simulink subsystem "GantryRobotSubsystem"  (R2024a)
settings: Solver=VariableStepAuto  StartTime=0.0  StopTime=10.0  RelTol=1e-3
model mask{DOF=3DOF, configAxis=XYZ, heightColumn=0.4, widthColumn=0.05, positionColumn1=[-0.5,-0.5,0], positionColumn2=[0.5,-0.5,0], positionColumn3=[-0.5,0.5,0], positionColumn4=[0.5,0.5,0], systemGuideX=Rail-block, strokeXMax=1, widthGuideX=0.05, diaScrewX=0.05, widthXMount=0.1, typeInertiaGuideX=Calculate from Geometry, densityGuideX=2700, massGuideX=0.1, COMGuideX=[0 0 0], MOIGuideX=[0.01 0.01 0.01], POIGuideX=[0 0 0], typeInertiaCarriageX=Calculate from Geometry, densityCarriageX=2700, massCarriageX=0.1, COMCarriageX=[0 0 0], MOICarriageX=[0.01 0.01 0.01], POICarriageX=[0 0 0], colorGuideX=[0.7 0.6 0.4], colorCarriageX=[0.5 0.5 0.9], systemGuideY=Rail-block, strokeYMax=1, widthGuideY=0.05, diaScrewY=0.05, widthYMount=0.05, typeInertiaGuideY=Calculate from Geometry, densityGuideY=2700, massGuideY=0.1, COMGuideY=[0 0 0], MOIGuideY=[0.01 0.01 0.01], POIGuideY=[0 0 0], typeInertiaCarriageY=Calculate from Geometry, densityCarriageY=2700, massCarriageY=0.1, COMCarriageY=[0 0 0], MOICarriageY=[0.01 0.01 0.01], POICarriageY=[0 0 0], colorGuideY=[0.7 0.6 0.4], colorCarriageY=[0.5 0.5 0.9], systemGuideZ=Rail-block, strokeZMax=1, widthGuideZ=0.05, diaScrewZ=0.05, shiftZAxisDown=0.02, widthZMount=0.05, typeInertiaGuideZ=Calculate from Geometry, densityGuideZ=2700, massGuideZ=0.1, COMGuideZ=[0 0 0], MOIGuideZ=[0.01 0.01 0.01], POIGuideZ=[0 0 0], typeInertiaCarriageZ=Calculate from Geometry, densityCarriageZ=2700, massCarriageZ=0.1, COMCarriageZ=[0 0 0], MOICarriageZ=[0.01 0.01 0.01], POICarriageZ=[0 0 0], colorGuideZ=[0.7 0.6 0.4], colorCarriageZ=[0.5 0.5 0.9]}
  mask prompts: DOF "Degrees of freedom"; configAxis "Axis configurations"; heightColumn "Column height (m)"; widthColumn "Column width (m)"; positionColumn1 "Column 1 position (m)"; positionColumn2 "Column 2 position (m)"; positionColumn3 "Column 3 position (m)"; positionColumn4 "Column 4 position (m)"; systemGuideX "Guide system"; strokeXMax "Maximum stroke (m)"; widthGuideX "Guide width (m)"; diaScrewX "Screw diameter (m)"; widthXMount "Mount width (m)"; typeInertiaGuideX "Inertia type"; densityGuideX "Density (kg/m^3)"; massGuideX "Mass (kg)"; COMGuideX "Center of mass (m)"; MOIGuideX "Moments of inertia (kg*m^2)"; POIGuideX "Products of inertia (kg*m^2)"; typeInertiaCarriageX "Inertia type"; densityCarriageX "Density (kg/m^3)"; massCarriageX "Mass (kg)"; COMCarriageX "Center of mass (m)"; MOICarriageX "Moments of inertia (kg*m^2)"; POICarriageX "Products of inertia (kg*m^2)"; colorGuideX "Linear guide color"; colorCarriageX "Carriage color"; systemGuideY "Guide system"; strokeYMax "Maximum stroke (m)"; widthGuideY "Guide width (m)"; diaScrewY "Screw diameter (m)"; widthYMount "Mount width (m)"; typeInertiaGuideY "Inertia type"; densityGuideY "Density (kg/m^3)"; massGuideY "Mass (kg)"; COMGuideY "Center of mass (m)"; MOIGuideY "Moments of inertia (kg*m^2)"; POIGuideY "Products of inertia (kg*m^2)"; typeInertiaCarriageY "Inertia type"; densityCarriageY "Density (kg/m^3)"; massCarriageY "Mass (kg)"; COMCarriageY "Center of mass (m)"; MOICarriageY "Moments of inertia (kg*m^2)"; POICarriageY "Products of inertia (kg*m^2)"; colorGuideY "Linear guide color"; colorCarriageY "Carriage color"; systemGuideZ "Guide system"; strokeZMax "Maximum stroke (m)"; widthGuideZ "Guide width (m)"; diaScrewZ "Screw diameter (m)"; shiftZAxisDown "Downward shift of Z-axis (m)"; widthZMount "Mount width (m)"; typeInertiaGuideZ "Inertia type"; densityGuideZ "Density (kg/m^3)"; massGuideZ "Mass (kg)"; COMGuideZ "Center of mass (m)"; MOIGuideZ "Moments of inertia (kg*m^2)"; POIGuideZ "Products of inertia (kg*m^2)"; typeInertiaCarriageZ "Inertia type"; densityCarriageZ "Density (kg/m^3)"; massCarriageZ "Mass (kg)"; COMCarriageZ "Center of mass (m)"; MOICarriageZ "Moments of inertia (kg*m^2)"; POICarriageZ "Products of inertia (kg*m^2)"; colorGuideZ "Linear guide color"; colorCarriageZ "Carriage color"
undefined symbols (not defined in the file): X, Y, Z
libraries: sm_lib x92, CartesianLib x46, nesl_utility x38
(part 4 of 4)

== system GantryRobotSubsystem/GantryRobotVariant/XYZR Gantry/Y-Axis Unit ==
  PS-Simulink Converter : nesl_utility/PS-Simulink Converter  PhysicalDomain=network_engine_domain  SubClassName=ps_output  LeftPortType=input  RightPortType=output  PseudoPeriodic=off  Frequencies=[]  VectorFormat=inherit  Unit=inherit  AffineConversion=off
  PS-Simulink Converter1 : nesl_utility/PS-Simulink Converter  PhysicalDomain=network_engine_domain  SubClassName=ps_output  LeftPortType=input  RightPortType=output  PseudoPeriodic=off  Frequencies=[]  VectorFormat=inherit  Unit=inherit  AffineConversion=off
  PS-Simulink Converter2 : nesl_utility/PS-Simulink Converter  PhysicalDomain=network_engine_domain  SubClassName=ps_output  LeftPortType=input  RightPortType=output  PseudoPeriodic=off  Frequencies=[]  VectorFormat=inherit  Unit=inherit  AffineConversion=off
  Prismatic Joint2 : sm_lib/Joints/Prismatic Joint  JointMode=Normal  CompositeWrenchDir=FollowerOnBase  CompositeWrenchFrame=BaseFrame  SenseConstraintForce=off  SenseConstraintTorque=off  SenseTotalForce=off  SenseTotalTorque=off  PositionTargetSpecify=off  PositionTargetPriority=High  PositionTargetValue=0  PositionTargetValueUnits=m  VelocityTargetSpecify=off  VelocityTargetPriority=High  VelocityTargetValue=0  VelocityTargetValueUnits=m/s  EquilibriumPosition=0  EquilibriumPositionUnits=m  SpringStiffness=0  SpringStiffnessUnits=N/m  DampingCoefficient=0  DampingCoefficientUnits=N/(m/s)  LowerLimitSpecify=on  LowerLimitBound=-0.5*strokeYMax  LowerLimitBoundUnits=m  LowerLimitStiffness=1e6  LowerLimitStiffnessUnits=N/m  LowerLimitDamping=1e3  LowerLimitDampingUnits=N/(m/s)  LowerLimitTransitionRegionWidth=1e-4  LowerLimitTransitionRegionWidthUnits=m  UpperLimitSpecify=on  UpperLimitBound=0.5*strokeYMax  UpperLimitBoundUnits=m  UpperLimitStiffness=1e6  UpperLimitStiffnessUnits=N/m  UpperLimitDamping=1e3  UpperLimitDampingUnits=N/(m/s)  UpperLimitTransitionRegionWidth=1e-4  UpperLimitTransitionRegionWidthUnits=m  TorqueActuationMode=InputTorque  MotionActuationMode=ComputedMotion  SensePosition=on  SenseVelocity=on  SenseAcceleration=on  SenseTorqueForce=off  SenseLowerLimitTorqueForce=off  SenseUpperLimitTorqueForce=off
  Rigid Transform1 : sm_lib/Frames and Transforms/Rigid Transform  RotationMethod=None  FollAlignAxisA=+X  BaseAlignAxisA=+Y  FollAlignAxisB=+Y  BaseAlignAxisB=+Z  RotationStandardAxis=+Z  RotationAngle=0  RotationAngleUnits=deg  RotationArbitraryAxis=[0 0 1]  RotationSequenceAxes=BaseAxes  RotationSequence=XYZ  RotationSequenceAngles=[0 0 0]  RotationSequenceAnglesUnits=deg  RotationMatrix=[1 0 0;0 1 0;0 0 1]  Quaternion=[1 0 0 0]  TranslationMethod=StandardAxis  TranslationCartesianOffset=[0 0 0]  TranslationCartesianOffsetUnits=m  TranslationStandardAxis=+Y  TranslationStandardOffset=-positionColumn1(2)  TranslationStandardOffsetUnits=m  TranslationROffset=0  TranslationROffsetUnits=m  TranslationThetaOffset=0  TranslationThetaOffsetUnits=deg  TranslationZOffset=0  TranslationZOffsetUnits=m
  Rigid Transform2 : sm_lib/Frames and Transforms/Rigid Transform  RotationMethod=None  FollAlignAxisA=+X  BaseAlignAxisA=+Y  FollAlignAxisB=+Y  BaseAlignAxisB=+Z  RotationStandardAxis=+Z  RotationAngle=0  RotationAngleUnits=deg  RotationArbitraryAxis=[0 0 1]  RotationSequenceAxes=BaseAxes  RotationSequence=XYZ  RotationSequenceAngles=[0 0 0]  RotationSequenceAnglesUnits=deg  RotationMatrix=[1 0 0;0 1 0;0 0 1]  Quaternion=[1 0 0 0]  TranslationMethod=StandardAxis  TranslationCartesianOffset=[0 0 0]  TranslationCartesianOffsetUnits=m  TranslationStandardAxis=+Y  TranslationStandardOffset=positionColumn2(2)  TranslationStandardOffsetUnits=m  TranslationROffset=0  TranslationROffsetUnits=m  TranslationThetaOffset=0  TranslationThetaOffsetUnits=deg  TranslationZOffset=0  TranslationZOffsetUnits=m
  Rigid Transform3 : sm_lib/Frames and Transforms/Rigid Transform  RotationMethod=StandardAxis  FollAlignAxisA=+X  BaseAlignAxisA=+Y  FollAlignAxisB=+Y  BaseAlignAxisB=+Z  RotationStandardAxis=+X  RotationAngle=-90  RotationAngleUnits=deg  RotationArbitraryAxis=[0 0 1]  RotationSequenceAxes=FollowerAxes  RotationSequence=XYX  RotationSequenceAngles=[0 0 0]  RotationSequenceAnglesUnits=deg  RotationMatrix=[1 0 0;0 1 0;0 0 1]  Quaternion=[1 0 0 0]  TranslationMethod=None  TranslationCartesianOffset=[0 0 0]  TranslationCartesianOffsetUnits=m  TranslationStandardAxis=+Z  TranslationStandardOffset=0  TranslationStandardOffsetUnits=m  TranslationROffset=0  TranslationROffsetUnits=m  TranslationThetaOffset=0  TranslationThetaOffsetUnits=deg  TranslationZOffset=0  TranslationZOffsetUnits=m
  Rigid Transform4 : sm_lib/Frames and Transforms/Rigid Transform  RotationMethod=StandardAxis  FollAlignAxisA=+X  BaseAlignAxisA=+Y  FollAlignAxisB=+Y  BaseAlignAxisB=+Z  RotationStandardAxis=+X  RotationAngle=90  RotationAngleUnits=deg  RotationArbitraryAxis=[0 0 1]  RotationSequenceAxes=FollowerAxes  RotationSequence=XYX  RotationSequenceAngles=[0 0 0]  RotationSequenceAnglesUnits=deg  RotationMatrix=[1 0 0;0 1 0;0 0 1]  Quaternion=[1 0 0 0]  TranslationMethod=None  TranslationCartesianOffset=[0 0 0]  TranslationCartesianOffsetUnits=m  TranslationStandardAxis=+Z  TranslationStandardOffset=0  TranslationStandardOffsetUnits=m  TranslationROffset=0  TranslationROffsetUnits=m  TranslationThetaOffset=0  TranslationThetaOffsetUnits=deg  TranslationZOffset=0  TranslationZOffsetUnits=m
  Y-Axis Linear Stage : CartesianLib/Linear Stage  systemGuide=Rail-block  axisGuide=Y-axis  stroke=1  widthRail=0.05  diaScrew=0.05  typeInertiaGuide=Calculate from Geometry  densityGuide=2700  massGuide=0.1  CMGuide=[0 0 0]  MOIGuide=[0.01 0.01 0.01]  POIGuide=[0 0 0]  typeInertiaCarriage=Calculate from Geometry  densityCarriage=2700  massCarriage=0.1  CMCarriage=[0 0 0]  MOICarriage=[0.01 0.01 0.01]  POICarriage=[0 0 0]  colorGuide=colorGuideY  colorCarriage=colorCarriageY
  YA : PMIOPort  Side=Left
  F : PMIOPort  Port=2  Side=Left
  B1 : PMIOPort  Port=3  Side=Right
  B2 : PMIOPort  Port=4  Side=Right
  Out Bus Element : Outport  PortName=YS  Element=Yp (m)
  BusElementOut : Outport  PortName=YS  Element=Yv (m/s)
  BusElementOut1 : Outport  PortName=YS  Element=Ya (m^2/s)
  wires:
  PS-Simulink Converter/1 -> Out Bus Element/1
  PS-Simulink Converter2/1 -> BusElementOut1/1
  PS-Simulink Converter1/1 -> BusElementOut/1
  connections:
  Prismatic Joint2/RConn4 -- PS-Simulink Converter2/LConn1
  Prismatic Joint2/RConn2 -- PS-Simulink Converter/LConn1
  Prismatic Joint2/RConn3 -- PS-Simulink Converter1/LConn1
  Rigid Transform2/LConn1 -- B2/RConn1
  F/RConn1 -- Y-Axis Linear Stage/LConn1
  Rigid Transform1/LConn1 -- B1/RConn1
  Prismatic Joint2/LConn2 -- YA/RConn1
  Y-Axis Linear Stage/RConn1 -- Rigid Transform2/RConn1 -- Rigid Transform1/RConn1
  Prismatic Joint2/RConn1 -- Rigid Transform4/LConn1
  Rigid Transform3/LConn1 -- Y-Axis Linear Stage/RConn2
  Rigid Transform4/RConn1 -- Y-Axis Linear Stage/LConn2
  Prismatic Joint2/LConn1 -- Rigid Transform3/RConn1

== system GantryRobotSubsystem/GantryRobotVariant/XYZR Gantry/Z-Axis Unit ==
  PS-Simulink Converter : nesl_utility/PS-Simulink Converter  PhysicalDomain=network_engine_domain  SubClassName=ps_output  LeftPortType=input  RightPortType=output  PseudoPeriodic=off  Frequencies=[]  VectorFormat=inherit  Unit=inherit  AffineConversion=off
  PS-Simulink Converter1 : nesl_utility/PS-Simulink Converter  PhysicalDomain=network_engine_domain  SubClassName=ps_output  LeftPortType=input  RightPortType=output  PseudoPeriodic=off  Frequencies=[]  VectorFormat=inherit  Unit=inherit  AffineConversion=off
  PS-Simulink Converter2 : nesl_utility/PS-Simulink Converter  PhysicalDomain=network_engine_domain  SubClassName=ps_output  LeftPortType=input  RightPortType=output  PseudoPeriodic=off  Frequencies=[]  VectorFormat=inherit  Unit=inherit  AffineConversion=off
  Prismatic Joint2 : sm_lib/Joints/Prismatic Joint  JointMode=Normal  CompositeWrenchDir=FollowerOnBase  CompositeWrenchFrame=BaseFrame  SenseConstraintForce=off  SenseConstraintTorque=off  SenseTotalForce=off  SenseTotalTorque=off  PositionTargetSpecify=off  PositionTargetPriority=High  PositionTargetValue=0  PositionTargetValueUnits=m  VelocityTargetSpecify=off  VelocityTargetPriority=High  VelocityTargetValue=0  VelocityTargetValueUnits=m/s  EquilibriumPosition=0  EquilibriumPositionUnits=m  SpringStiffness=0  SpringStiffnessUnits=N/m  DampingCoefficient=0  DampingCoefficientUnits=N/(m/s)  LowerLimitSpecify=on  LowerLimitBound=-0.5*strokeZMax  LowerLimitBoundUnits=m  LowerLimitStiffness=1e6  LowerLimitStiffnessUnits=N/m  LowerLimitDamping=1e3  LowerLimitDampingUnits=N/(m/s)  LowerLimitTransitionRegionWidth=1e-4  LowerLimitTransitionRegionWidthUnits=m  UpperLimitSpecify=on  UpperLimitBound=0.5*strokeZMax  UpperLimitBoundUnits=m  UpperLimitStiffness=1e6  UpperLimitStiffnessUnits=N/m  UpperLimitDamping=1e3  UpperLimitDampingUnits=N/(m/s)  UpperLimitTransitionRegionWidth=1e-4  UpperLimitTransitionRegionWidthUnits=m  TorqueActuationMode=InputTorque  MotionActuationMode=ComputedMotion  SensePosition=on  SenseVelocity=on  SenseAcceleration=on  SenseTorqueForce=off  SenseLowerLimitTorqueForce=off  SenseUpperLimitTorqueForce=off
  Rigid Transform1 : sm_lib/Frames and Transforms/Rigid Transform  RotationMethod=None  FollAlignAxisA=+X  BaseAlignAxisA=+Y  FollAlignAxisB=+Y  BaseAlignAxisB=+Z  RotationStandardAxis=+Z  RotationAngle=0  RotationAngleUnits=deg  RotationArbitraryAxis=[0 0 1]  RotationSequenceAxes=BaseAxes  RotationSequence=XYZ  RotationSequenceAngles=[0 0 0]  RotationSequenceAnglesUnits=deg  RotationMatrix=[1 0 0;0 1 0;0 0 1]  Quaternion=[1 0 0 0]  TranslationMethod=StandardAxis  TranslationCartesianOffset=[0 0 0]  TranslationCartesianOffsetUnits=m  TranslationStandardAxis=+Z  TranslationStandardOffset=shiftZAxisDown  TranslationStandardOffsetUnits=m  TranslationROffset=0  TranslationROffsetUnits=m  TranslationThetaOffset=0  TranslationThetaOffsetUnits=deg  TranslationZOffset=0  TranslationZOffsetUnits=m
  Rigid Transform2 : sm_lib/Frames and Transforms/Rigid Transform  RotationMethod=None  FollAlignAxisA=+X  BaseAlignAxisA=+Y  FollAlignAxisB=+Y  BaseAlignAxisB=+Z  RotationStandardAxis=+X  RotationAngle=0  RotationAngleUnits=deg  RotationArbitraryAxis=[0 0 1]  RotationSequenceAxes=FollowerAxes  RotationSequence=XYX  RotationSequenceAngles=[0 0 0]  RotationSequenceAnglesUnits=deg  RotationMatrix=[1 0 0;0 1 0;0 0 1]  Quaternion=[1 0 0 0]  TranslationMethod=None  TranslationCartesianOffset=[0 0 0]  TranslationCartesianOffsetUnits=m  TranslationStandardAxis=+Z  TranslationStandardOffset=0  TranslationStandardOffsetUnits=m  TranslationROffset=0  TranslationROffsetUnits=m  TranslationThetaOffset=0  TranslationThetaOffsetUnits=deg  TranslationZOffset=0  TranslationZOffsetUnits=m
  Rigid Transform3 : sm_lib/Frames and Transforms/Rigid Transform  RotationMethod=None  FollAlignAxisA=+X  BaseAlignAxisA=+Y  FollAlignAxisB=+Y  BaseAlignAxisB=+Z  RotationStandardAxis=+X  RotationAngle=0  RotationAngleUnits=deg  RotationArbitraryAxis=[0 0 1]  RotationSequenceAxes=FollowerAxes  RotationSequence=XYX  RotationSequenceAngles=[0 0 0]  RotationSequenceAnglesUnits=deg  RotationMatrix=[1 0 0;0 1 0;0 0 1]  Quaternion=[1 0 0 0]  TranslationMethod=None  TranslationCartesianOffset=[0 0 0]  TranslationCartesianOffsetUnits=m  TranslationStandardAxis=+Z  TranslationStandardOffset=0  TranslationStandardOffsetUnits=m  TranslationROffset=0  TranslationROffsetUnits=m  TranslationThetaOffset=0  TranslationThetaOffsetUnits=deg  TranslationZOffset=0  TranslationZOffsetUnits=m
  Z-Axis Linear Stage : CartesianLib/Linear Stage  systemGuide=Rail-block  axisGuide=Z-axis  stroke=1  widthRail=0.05  diaScrew=0.05  typeInertiaGuide=Calculate from Geometry  densityGuide=2700  massGuide=0.1  CMGuide=[0 0 0]  MOIGuide=[0.01 0.01 0.01]  POIGuide=[0 0 0]  typeInertiaCarriage=Calculate from Geometry  densityCarriage=2700  massCarriage=0.1  CMCarriage=[0 0 0]  MOICarriage=[0.01 0.01 0.01]  POICarriage=[0 0 0]  colorGuide=colorGuideZ  colorCarriage=colorCarriageZ
  ZA : PMIOPort  Side=Left
  F : PMIOPort  Port=2  Side=Left
  B : PMIOPort  Port=3  Side=Right
  Out Bus Element : Outport  PortName=ZS  Element=Zp (m)
  BusElementOut : Outport  PortName=ZS  Element=Zv (m/s)
  BusElementOut1 : Outport  PortName=ZS  Element=Za (m^2/s)
  wires:
  PS-Simulink Converter/1 -> Out Bus Element/1
  PS-Simulink Converter2/1 -> BusElementOut1/1
  PS-Simulink Converter1/1 -> BusElementOut/1
  connections:
  Prismatic Joint2/RConn3 -- PS-Simulink Converter1/LConn1
  Prismatic Joint2/RConn2 -- PS-Simulink Converter/LConn1
  Prismatic Joint2/RConn4 -- PS-Simulink Converter2/LConn1
  F/RConn1 -- Z-Axis Linear Stage/LConn1
  Rigid Transform1/LConn1 -- B/RConn1
  Prismatic Joint2/LConn2 -- ZA/RConn1
  Rigid Transform1/RConn1 -- Z-Axis Linear Stage/RConn1
  Prismatic Joint2/RConn1 -- Rigid Transform3/LConn1
  Rigid Transform2/LConn1 -- Z-Axis Linear Stage/RConn2
  Rigid Transform3/RConn1 -- Z-Axis Linear Stage/LConn2
  Prismatic Joint2/LConn1 -- Rigid Transform2/RConn1
